simulink model "hpfbuttter2nd"  (R2026a)
settings: Solver=ode8  StopTime=2  FixedStep=1e-3
undefined symbols (not defined in the file): dspblkCoreblockFVToolHelper, gcbh
libraries: simulink x1
settings Model: Creator=auralius  LastModifiedBy=auralius

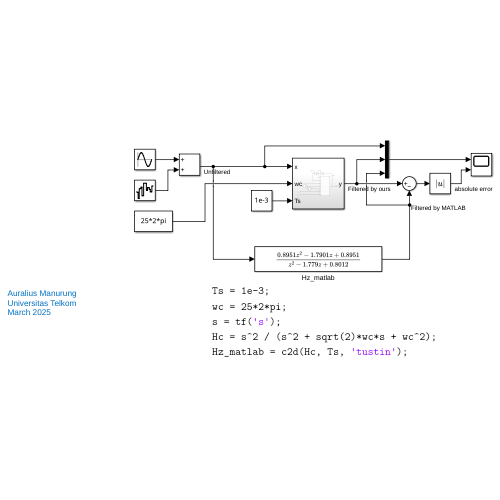
[thumbnail: Simulink's stored preview of the top-level diagram]
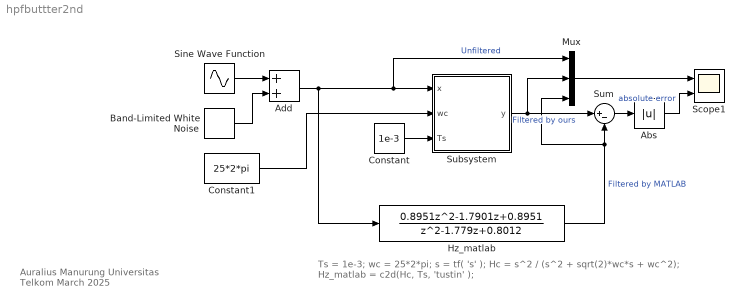
== system hpfbuttter2nd ==
  note: Ts = 1e-3;
      | wc = 25*2*pi;
      | s = tf( 's' );
      | Hc = s^2 / (s^2 + sqrt(2)*wc*s + wc^2);
      | Hz_matlab = c2d(Hc, Ts, 'tustin' );
  note: Auralius Manurung
      | Universitas Telkom
      | March 2025
  Abs : Abs  SaturateOnIntegerOverflow=off
  Add : Sum
  Band-Limited White Noise : simulink/Sources/Band-Limited White Noise  Cov=[0.1]  Ts=1e-3  seed=[23341]
  Constant : Constant  Value=1e-3
  Constant1 : Constant  Value=25*2*pi
  Hz_matlab : DiscreteTransferFcn  LoadFcn=dspblkCoreblockFVToolHelper(gcbh,'load');  Numerator=[0.8951 -1.7901 0.8951]  Denominator=[1 -1.779 0.8012]
      settings: CopyFcn=dspblkCoreblockFVToolHelper(gcbh,'copy');  DeleteFcn=dspblkCoreblockFVToolHelper(gcbh,'close');  ModelCloseFcn=dspblkCoreblockFVToolHelper(gcbh,'close');  PreSaveFcn=dspblkCoreblockFVToolHelper(gcbh,'presave');  PostSaveFcn=dspblkCoreblockFVToolHelper(gcbh,'postsave');  CloseFcn=dspblkCoreblockFVToolHelper(gcbh,'close');
  Mux : Mux  Inputs=3
  Scope1 : Scope  NumInputPorts=2
      settings: ActiveDisplayYMinimum=-46.666756965780117  ActiveDisplayYMaximum=51.392818465111787
  Sine Wave Function : Sin  Frequency=50*pi  SampleTime=0
  Subsystem : Subsystem
  Sum : Sum  Inputs=|+-
  wires:
  Constant/1 -> Subsystem/3(Ts)
  Sine Wave Function/1 -> Add/1
  Band-Limited White Noise/1 -> Add/2
  Constant1/1 -> Subsystem/2(wc)
  Add/1 -> Hz_matlab/1, Mux/1, Subsystem/1(x)  "Unfiltered"
  Subsystem/1(y) -> Sum/1, Mux/2  "Filtered by ours"
  Hz_matlab/1 -> Mux/3, Sum/2  "Filtered by MATLAB"
  Sum/1 -> Abs/1
  Abs/1 -> Scope1/2  "absolute error"
  Mux/1 -> Scope1/1

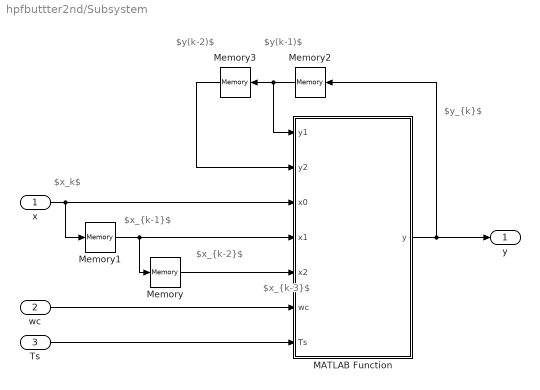
== system hpfbuttter2nd/Subsystem ==
  note: $x_k$
  note: $x_{k-2}$
  note: $x_{k-1}$
  note: $y_{k}$
  note: $y(k-2)$
  note: $y(k-1)$
  note: $x_{k-3}$
  x : Inport
  wc : Inport  Port=2
  Ts : Inport  Port=3
  MATLAB Function : MATLAB Function  TreatAsAtomicUnit=on
  Memory{,1..3} (4 alike) : Memory  InheritSampleTime=on
  y : Outport
  wires:
  wc/1 -> MATLAB Function/6(wc)
  MATLAB Function/1(y) -> y/1, Memory2/1
  Memory2/1 -> MATLAB Function/1(y1), Memory3/1
  Ts/1 -> MATLAB Function/7(Ts)
  Memory1/1 -> MATLAB Function/4(x1), Memory/1
  Memory/1 -> MATLAB Function/5(x2)
  x/1 -> Memory1/1, MATLAB Function/3(x0)
  Memory3/1 -> MATLAB Function/2(y2)

== matlab function hpfbuttter2nd/Subsystem/MATLAB Function ==
  data: y1 input; y2 input; x0 input; x1 input; x2 input; y output; wc input; Ts input
function y = HPF(y1, y2, x0, x1, x2, wc, Ts)
% Second-order Butterworth high-pass filter
%
% y1 = y(k-1)
% y2 = y(k-2)
% x0 = x(k)
% x1 = x(k-1)
% x2 = x(k-2)
% wc = cutoff angular frequency [rad/s]
% Ts = sampling period [s]

sq22 = 2*sqrt(2);
Tswc = Ts * wc;

A = 1 + sq22/Tswc + 4/Tswc^2;
B = 2 - 8/Tswc^2;
C = 1 - sq22/Tswc + 4/Tswc^2;
D = 4/Tswc^2;

y = (D*(x0 - 2*x1 + x2) - B*y1 - C*y2) / A;
end
